simulink model "PM_DDD_ref"  (R2024b)
settings: Solver=ode1  StartTime=0.0  StopTime=10.0  FixedStep=0.0005  RelTol=1e-3
libraries: Libs_second x5
settings Model: DataDictionary=PM_DDD_dd.sldd  EnableAccessToBaseWorkspace=off  Creator=wai484  LastModifiedBy=wai484
settings DataIOCC: SaveOutput=off  SignalLogging=off  DSMLogging=off  StreamToWks=off  SaveTime=off  ReturnWorkspaceOutputs=off
settings OptimizationCC: StateBitsets=on  DataBitsets=on  EfficientFloat2IntCast=on
settings DebuggingCC: ConsistencyChecking=error  SignalInfNanChecking=warning  ReadBeforeWriteMsg=EnableAllAsError  WriteAfterWriteMsg=EnableAllAsError  WriteAfterReadMsg=EnableAllAsError  AlgebraicLoopMsg=error  ArtificialAlgebraicLoopMsg=error  SaveWithDisabledLinksMsg=error  SaveWithParameterizedLinksMsg=error  BlockPriorityViolationMsg=error  TimeAdjustmentMsg=warning  SolverPrmCheckMsg=error  InheritedTsInSrcMsg=error  SingleTaskRateTransMsg=error  TasksWithSamePriorityMsg=error  SigSpecEnsureSampleTimeMsg=error  CheckMatrixSingularityMsg=error  IntegerOverflowMsg=error  ParameterUnderflowMsg=error  ParameterPrecisionLossMsg=error  ParameterTunabilityLossMsg=error  FixptConstUnderflowMsg=error  FixptConstOverflowMsg=error  FixptConstPrecisionLossMsg=error  UnderSpecifiedDataTypeMsg=error  UnnecessaryDatatypeConvMsg=warning  VectorMatrixConversionMsg=error  UnconnectedInputMsg=error  UnconnectedOutputMsg=error  UnconnectedLineMsg=error  SFcnCompatibilityMsg=error  UniqueDataStoreMsg=error  BusObjectLabelMismatch=error  RootOutportRequireBusObject=error  AssertControl=DisableAll  ModelReferenceIOMismatchMessage=error  UnknownTsInhSupMsg=error  ModelReferenceDataLoggingMessage=error  ModelReferenceNoExplicitFinalValueMsg=error  StateNameClashWarn=warning  OperatingPointInterfaceChecksumMismatchMsg=error  StrictBusMsg=ErrorOnBusTreatedAsVector  NonBusSignalsTreatedAsBus=error  SFUnusedDataAndEventsDiag=error  SFInvalidInputDataAccessInChartInitDiag=error  SFTransitionOutsideNaturalParentDiag=error  SFUnreachableExecutionPathDiag=error  SFUndirectedBroadcastEventsDiag=error  SFTransitionActionBeforeConditionDiag=error  SFTemporalDelaySmallerThanSampleTimeDiag=error  SFSelfTransitionDiag=error  SFExecutionAtInitializationDiag=error  IntegerSaturationMsg=error  ForceCombineOutputUpdateInSim=on  UnderSpecifiedDimensionMsg=error  VariantConditionMismatch=error  InheritVATfromSVC=error  VariantConfigNotUsedByTopModel=error  ParamWriterValidationControl=DisableAll
settings ModelReferenceCC: EnableParallelModelReferenceBuilds=on
settings SFSimCC: CompileTimeRecursionLimit=0  EnableRuntimeRecursion=off  MATLABDynamicMemAlloc=off
settings CodeAppCC: ForceParamTrailComments=on  StateflowObjectComments=on  MATLABSourceComments=on
settings GRTTargetCC: UtilityFuncGeneration=Shared location  SupportNonFinite=off  OptimizeReductions=on

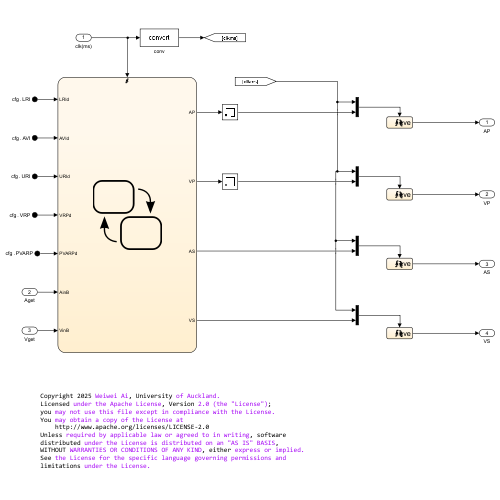
[thumbnail: Simulink's stored preview of the top-level diagram]
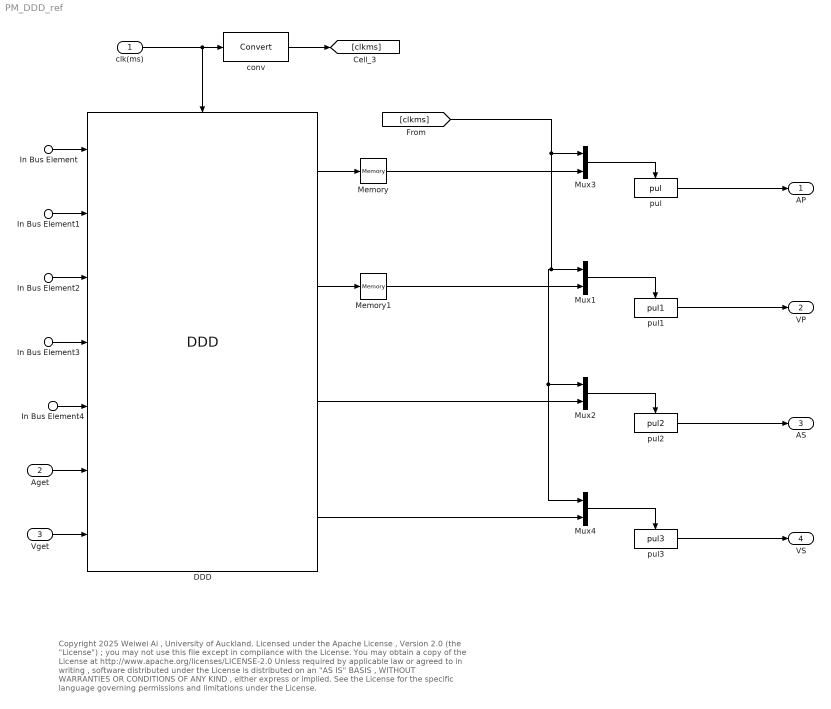
== system PM_DDD_ref ==
  note: Copyright 2025 Weiwei Ai , University of Auckland.
      | Licensed under the Apache License , Version 2.0 (the "License") ;
      | you may not use this file except in compliance with the License.
      | You may obtain a copy of the License at
      | http://www.apache.org/licenses/LICENSE-2.0
      | Unless required by applicable law or agreed to in writing , software
      | distributed under the License is distributed on an "AS IS" BASIS ,
      | WITHOUT WARRANTIES OR CONDITIONS OF ANY KIND , either express or implied.
      | See the License for the specific language governing permissions and
      | limitations under the License.
  clk(ms) : Inport
  Aget : Inport  Port=2
  Vget : Inport  Port=3
  In Bus Element : Inport  Port=4  PortName=cfg  Element=LRI
  In Bus Element1 : Inport  Port=4  PortName=cfg  Element=AVI
  In Bus Element2 : Inport  Port=4  PortName=cfg  Element=URI
  In Bus Element3 : Inport  Port=4  PortName=cfg  Element=VRP
  In Bus Element4 : Inport  Port=4  PortName=cfg  Element=PVARP
  DDD : Libs_second/PM_DDD_v3/DDD  SystemSampleTime=-1  VariantActivationTime=update diagram  AllowFlexibleInterface=on  Latency=0  AutoFrameSizeCalculation=off
  Memory : Memory
  Memory1 : Memory
  Mux{1..4} (4 alike) : Mux  Inputs=2
  conv : DataTypeConversion  SaturateOnIntegerOverflow=off  RndMeth=Floor
  pul : Libs_second/PM_DDD_v3/pul  SystemSampleTime=-1  VariantActivationTime=update diagram  AllowFlexibleInterface=on  Latency=0  AutoFrameSizeCalculation=off
  pul1 : Libs_second/PM_DDD_v3/pul1  SystemSampleTime=-1  VariantActivationTime=update diagram  AllowFlexibleInterface=on  Latency=0  AutoFrameSizeCalculation=off
  pul2 : Libs_second/PM_DDD_v3/pul2  SystemSampleTime=-1  VariantActivationTime=update diagram  AllowFlexibleInterface=on  Latency=0  AutoFrameSizeCalculation=off
  pul3 : Libs_second/PM_DDD_v3/pul3  SystemSampleTime=-1  VariantActivationTime=update diagram  AllowFlexibleInterface=on  Latency=0  AutoFrameSizeCalculation=off
  AP : Outport
  VP : Outport  Port=2
  AS : Outport  Port=3
  VS : Outport  Port=4
  wires:
  Mux2/1 -> pul2/Trigger
  Vget/1 -> DDD/7
  conv/1 -> [clkms]
  [clkms] -> Mux4/1, Mux2/1, Mux1/1, Mux3/1
  pul1/1 -> VP/1
  Mux1/1 -> pul1/Trigger
  DDD/2 -> Memory1/1
  Memory/1 -> Mux3/2
  Memory1/1 -> Mux1/2
  DDD/4 -> Mux4/2
  pul/1 -> AP/1
  pul3/1 -> VS/1
  pul2/1 -> AS/1
  Mux3/1 -> pul/Trigger
  Mux4/1 -> pul3/Trigger
  clk(ms)/1 -> conv/1, DDD/Trigger
  Aget/1 -> DDD/6
  DDD/3 -> Mux2/2
  DDD/1 -> Memory/1
  In Bus Element/1 -> DDD/1
  In Bus Element1/1 -> DDD/2
  In Bus Element2/1 -> DDD/3
  In Bus Element3/1 -> DDD/4
  In Bus Element4/1 -> DDD/5
